simulink model "Hardware_testng_simulink_both"  (R2024b)
settings: Solver=ode1  StartTime=0.0  StopTime=15  FixedStep=0.005  RelTol=1e-3  EnableMultiTasking=on
undefined symbols (not defined in the file or in its folder): DiscIntNeverNeededParam, initialPose, maxAngularAcc, maxAngularVel, maxLinearAcc, maxLinearVel, poseTol, Ts, wps1
libraries: simulink_extras x12, stmnucleolib x12, simulink x4, hdlsllib x1, embmathops x1, robotcorelib x1
(part 1 of 2)
settings Model: ExtModeTrigDuration=10  Creator=ASUS  LastModifiedBy=Chhay
settings OptimizationCC: EnhancedBackFolding=on  PassReuseOutputArgsAs=Individual arguments  ZeroExternalMemoryAtStartup=off  ZeroInternalMemoryAtStartup=off  MaxStackSize=64  OptimizeBlockOrder=speed  DifferentSizesBufferReuse=on  OptimizationCustomize=off  EfficientTunableParamExpr=on
settings DebuggingCC: ParameterTunabilityLossMsg=error
settings HardwareCC: ProdBitPerPointer=32  ProdBitPerSizeT=32  ProdBitPerPtrDiffT=32  ProdLargestAtomicInteger=Long  ProdLargestAtomicFloat=Double  ProdWordSize=32  ProdLongLongMode=on  ProdHWDeviceType=ARM Compatible->ARM Cortex
settings SFSimCC: MATLABDynamicMemAlloc=off
settings RTWCC: Description=Embedded Coder  SystemTargetFile=ert.tlc  HardwareBoard=STM32 Nucleo H743ZI2  TemplateMakefile=ert_default_tmf  Toolchain=GNU Tools for ARM Embedded Processors  GPUComputeCapability=3.5
settings CodeAppCC: ForceParamTrailComments=on  IgnoreCustomStorageClasses=off  OperatorAnnotations=on  SimulinkDataObjDesc=on  SFDataObjDesc=on  InsertBlockDesc=on
settings ERTTargetCC: SupportContinuousTime=on  SupportVariableSizeSignals=on  ExtModeTransport=3  ExtModeStaticAlloc=on  ExtModeStaticAllocSize=2000  ExtModeMexFile=ext_xcp  ExtModeMexArgs=1 6 115200  ExtModeIntrfLevel=Level2 - Open  InlinedParameterPlacement=Hierarchical  RootIOFormat=Structure reference  DynamicArrayContainerType=coder::array

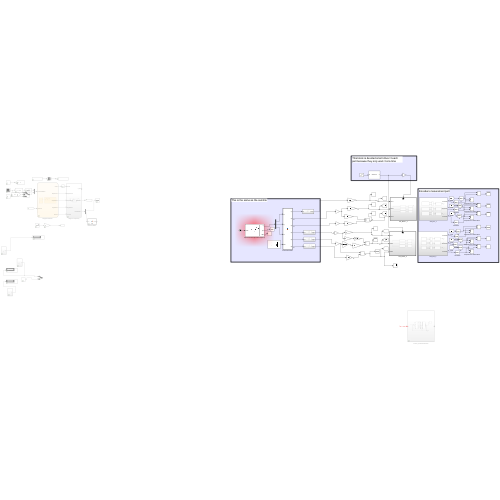
[thumbnail: Simulink's stored preview of the top-level diagram]
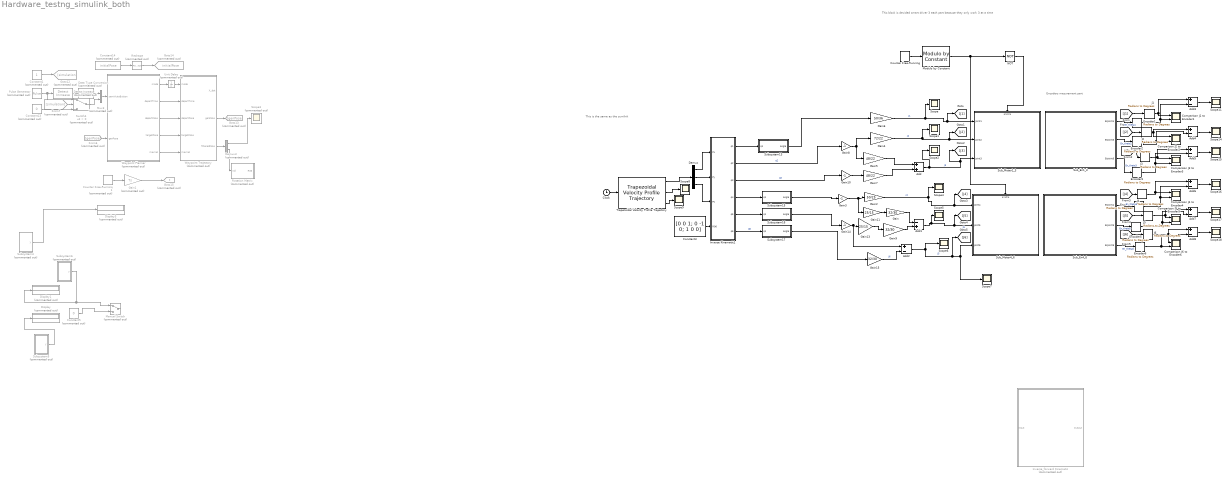
== system Hardware_testng_simulink_both ==
  note: Encoders mesurement part
  note: This block is devided smart driver 3 each part because they only work 3 at a time
  note: This is the same as the sumlink
  Add : Sum
  Add1 : Sum  Inputs=-+
  Add{2..8} (7 alike) : Sum  Inputs=+-
  Clock : Clock
  Comparison J1 to Encoder1 : Scope  NumInputPorts=2
  Comparison J2 to Encoder2 : Scope  NumInputPorts=2
  Comparison J3 to Encoder3 : Scope  NumInputPorts=2
  Comparison J4 to Encoder4 : Scope  NumInputPorts=2
  Comparison J5 to Encoder5 : Scope  NumInputPorts=2
  Comparison J6 to Encoder6 : Scope  NumInputPorts=2
  Constant1 : Constant  Commented=on
  Constant13 : Constant  Commented=on  Value=0
  Constant14 : Constant  Commented=on  Value=initialPose
  Constant3 : Constant  Value=[0 0 1; 0 -1 0; 1 0 0]
  Constant5 : Constant  Commented=on  Value=0
  Counter Free-Running : hdlsllib/Sources/Counter Free-Running  NumBits=16  tsamp=-1
  Counter Free-Running1 : simulink/Sources/Counter Free-Running  Commented=on  NumBits=16  tsamp=-1
  Data Type Conversion : DataTypeConversion  Commented=on  OutDataTypeStr=double  SaturateOnIntegerOverflow=off  RndMeth=Floor
  Demux : Demux  Outputs=3
  Demux3 : Demux  Commented=on  Outputs=[3,1]
  Detect Increase : simulink/Logic and Bit Operations/Detect Increase  Commented=on  vinit=0.0  OutDataTypeStr=boolean
  Display : Display  Commented=on
  Display1 : Display  Commented=on
  Display3 : Display  Commented=on
  Encoder{1..6} (6 alike) : simulink_extras/Transformations/Radians to Degrees
  From6 : From  Commented=on  GotoTag=genPose
  From7 : From  Commented=on  GotoTag=simulation
  Gain : Gain  Gain=32/30
  Gain1 : Gain  Commented=on  Gain=Ts  OutDataTypeStr=double
  Gain{3,8,10,14} (4 alike) : Gain  Gain=-1
  Gain11 : Gain  Gain=25/15
  Gain13 : Gain  Gain=25/15
  Gain15 : Gain  Gain=32/30
  Gain2 : Gain  Gain=50/25
  Gain4 : Gain  Gain=72/22
  Gain5 : Gain  Gain=48/22
  Gain6 : Gain  Gain=50/36  OutDataTypeStr=Inherit: Same as input
  Gain7 : Gain  Gain=48/22
  Gain9 : Gain  Gain=32/30
  Goto12 : Goto  Commented=on  GotoTag=simulation
  Goto13 : Goto  Commented=on  GotoTag=genPose
  Goto14 : Goto  Commented=on  GotoTag=initialPose  TagVisibility=global
  Goto15 : Goto  Commented=on  GotoTag=t  TagVisibility=global
  Inverse Kinematic1 : MATLAB Function  TreatAsAtomicUnit=on
  Inverse_forward Kinematic : Subsystem  Commented=on
  J{1..6} (6 alike) : simulink_extras/Transformations/Radians to Degrees
  Manual Switch : ManualSwitch  Commented=on
  Modulo by Constant : embmathops/Modulo by Constant  Denominator=2  SimulateUsing=Code generation
      settings: LibrarySourceBlock=embeddedMathLib/Modulo by Constant
  Mux3 : Mux  Commented=on  Inputs=2
  NOT : Logic  Operator=NOT  IconShape=distinctive  AllPortsSameDT=off  OutDataTypeStr=boolean
  Pulse Generator : DiscretePulseGenerator  Commented=on  PulseType=Time based  Period=30  PulseWidth=5  PhaseDelay=5
  Reshape : Reshape  Commented=on  OutputDimensionality=Column vector (2-D)
  Rotation Matrix : MATLAB Function  Commented=on  TreatAsAtomicUnit=on
  Scope{,1..2,4..9,11,14..18} (15 alike) : Scope
  Scope3 : Scope  Commented=on
  Sub_En1_3 : Subsystem
  Sub_En4_6 : Subsystem
  Sub_Moter1_3 : Subsystem
  Sub_Moter4_6 : Subsystem
  Subsystem13 : Subsystem
  Subsystem15 : Subsystem
  Subsystem16 : Subsystem
  Subsystem17 : Subsystem
  Subsystem4 : Subsystem  Commented=on
  Subsystem5 : Subsystem  Commented=on
  Subsystem6 : Subsystem  Commented=on
  Switch4 : Switch  Commented=on  Criteria=u2 > Threshold  SaturateOnIntegerOverflow=off  InputSameDT=off
  Trapezoidal Velocity Profile Trajectory : robotcorelib/Trapezoidal Velocity Profile Trajectory  WaypointSource=Internal  Waypoints=Way4  NumParams=1  Parameter1=End Time  Parameter2=End Time  ParameterSource=Internal  PeakVelocity=[ 2; 2 ]  Acceleration=[ 1; 2 ]  EndTime=2  AccelTime=[ 1; 2 ]  SimulateUsing=Interpreted execution
  Unit Delay : UnitDelay  Commented=on  SampleTime=-1  HasFrameUpgradeWarning=on
  Waypoint Planner : Stateflow chart  Commented=on  TreatAsAtomicUnit=on
      settings: PortSchema="{\"entries\":[{\"content\":{\"sides\":[{\"content\":{\"connectorIds\":[\"In2\",\"In1\"]},\"type\":\"ConnectorPlacement.EquallySpacedRectSide\",\"uuid\":\"2f7816bf-e041-4d80-a35c-f5abf025ca4f\"},{\"content\":{\"connectorIds\":[\"Out5\",\"Out1\",\"Out2\",\"Out3\",\"Out4\"],\"side\":\"RIGHT\"},\"type\":\"ConnectorPlacement.EquallySpacedRectSide\",\"uuid\":\"030a9877-c717-421f-9736-0adf27f6f35f\"},{\"content\":{\"side\":\"TOP\"},\"type\":\"ConnectorPlacement.EquallySpacedRectSide\",\"uuid\":\"ba023d22-bb45-4b84-a72f-1110f01393be\"}]},\"type\":\"ConnectorPlacement.EquallySpacedConnector\",\"uuid\":\"d2a85391-dfa2-4741-8917-4ca0c8ef44a5\"}],\"packageUris\":[\"http://schema.mathworks.com/mf0/Connector/R2020b\"],\"version\":\"1.0\"}"
  Waypoint Trajectory : Subsystem  Commented=on
  wires:
  Counter Free-Running/1 -> Modulo by Constant/1
  Modulo by Constant/1 -> NOT/1, Sub_Moter4_6/Enable
  NOT/1 -> Sub_Moter1_3/Enable
  Gain/1 -> Add1/1
  Gain2/1 -> [J4], Sub_Moter4_6/1(joint4), Scope4/1  "J4"
  Gain6/1 -> Scope/1, Sub_Moter1_3/1(Joint1), [J1]  "J1"
  Gain5/1 -> Add/1
  Gain7/1 -> Add/2
  Sub_En1_3/1(EnJoint4) -> Encoder1/1  "En_theta1"
  Sub_En1_3/2(EnJoint5) -> Encoder2/1  "En_theta2"
  Sub_En1_3/3(EnJoint6) -> Encoder3/1  "En_theta3"
  Sub_En4_6/2(EnJoint5) -> Encoder5/1  "En_theta5"
  Sub_En4_6/3(EnJoint6) -> Encoder6/1  "En_theta6"
  Gain4/1 -> Sub_Moter1_3/2(Joint2), [J2], Scope1/1  "J2"
  Gain15/1 -> Add2/2  "J6"
  Gain13/1 -> Gain9/1
  Add/1 -> Sub_Moter1_3/3(Joint3), [J3], Scope2/1  "J3"
  Add1/1 -> Scope5/1, [J5], Sub_Moter4_6/2(Joint5)  "J5"
  Gain9/1 -> Add1/2
  Gain11/1 -> Gain/1
  [J1] -> J1/1
  [J2] -> J2/1
  [J3] -> J3/1
  [J5] -> J5/1
  [J6] -> J6/1
  [J4] -> J4/1
  Sub_En4_6/1(EnJoint4) -> Encoder4/1  "En_theta3"
  Add3/1 -> Scope11/1
  Add4/1 -> Scope14/1
  Add5/1 -> Scope15/1
  Add6/1 -> Scope16/1
  Add7/1 -> Scope17/1
  Add8/1 -> Scope18/1
  Gain14/1 -> Add2/1, Gain13/1
  Gain8/1 -> Gain5/1, Gain4/1
  Gain10/1 -> Gain7/1
  Subsystem16/1(angle) -> Gain14/1
  Subsystem13/1(angle) -> Gain6/1
  Subsystem15/1(angle) -> Gain3/1
  Encoder6/1 -> Add8/2, Comparison J6 to Encoder6/2
  J6/1 -> Add8/1, Comparison J6 to Encoder6/1
  Encoder5/1 -> Add7/2, Comparison J5 to Encoder5/2
  J5/1 -> Add7/1, Comparison J5 to Encoder5/1
  Encoder4/1 -> Add6/2, Comparison J4 to Encoder4/2
  J4/1 -> Add6/1, Comparison J4 to Encoder4/1
  Encoder3/1 -> Add5/2, Comparison J3 to Encoder3/2
  J3/1 -> Add5/1, Comparison J3 to Encoder3/1
  Encoder2/1 -> Add4/2, Comparison J2 to Encoder2/2
  J2/1 -> Comparison J2 to Encoder2/1, Add4/1
  Encoder1/1 -> Add3/2, Comparison J1 to Encoder1/2
  J1/1 -> Comparison J1 to Encoder1/1, Add3/1
  Subsystem17/1(angle) -> Gain15/1
  Add2/1 -> Scope6/1, Scope7/1, Sub_Moter4_6/3(Joint6), [J6]  "J5"
  Switch4/1 -> Mux3/2
  Unit Delay/1 -> Waypoint Trajectory/1(mode)
  Waypoint Trajectory/3(filteredPose) -> Demux3/1
  Reshape/1 -> Goto14/1
  From7/1 -> Switch4/2
  Waypoint Planner/2(departPose) -> Waypoint Trajectory/3(departPose)
  Demux3/1 -> Scope3/1
  Waypoint Trajectory/2(genPose) -> Goto13/1
  Waypoint Planner/3(targetPose) -> Waypoint Trajectory/4(targetPose)
  Constant13/1 -> Switch4/3
  Waypoint Planner/5(mode) -> Unit Delay/1
  Counter Free-Running1/1 -> Gain1/1
  Data Type Conversion/1 -> Mux3/1
  Waypoint Planner/1(departTime) -> Waypoint Trajectory/2(departTime)
  Inverse Kinematic1/6(q6) -> Subsystem17/1(q1)  "q6"
  Detect Increase/1 -> Data Type Conversion/1
  Demux3/2 -> Rotation Matrix/1(roll)
  Gain1/1 -> Goto15/1
  Constant1/1 -> Goto12/1
  From6/1 -> Waypoint Planner/1(genPose)
  Inverse Kinematic1/2(q2) -> Gain8/1  "q2"
  Constant14/1 -> Reshape/1
  Inverse Kinematic1/4(q4) -> Subsystem15/1(q1)
  Pulse Generator/1 -> Switch4/1, Detect Increase/1
  Inverse Kinematic1/5(q5) -> Subsystem16/1(q1)
  Inverse Kinematic1/1(q1) -> Subsystem13/1(q1)
  Mux3/1 -> Waypoint Planner/2(semiAutoButton)
  Inverse Kinematic1/3(q3) -> Gain10/1  "q3"
  Waypoint Planner/4(maxVel) -> Waypoint Trajectory/5(maxVel)
  ? -> Inverse_forward Kinematic/1(Input)
  Gain3/1 -> Gain11/1, Gain2/1
  Constant3/1 -> Inverse Kinematic1/4(R06)
  Trapezoidal Velocity Profile Trajectory/1 -> Demux/1
  Clock/1 -> Trapezoidal Velocity Profile Trajectory/1
  Subsystem4/1(y) -> Display3/1
  Subsystem5/1(y) -> Display/1
  Demux/1 -> Inverse Kinematic1/1(Px)
  Constant5/1 -> Manual Switch/2
  Subsystem6/1(y) -> Manual Switch/1, Display1/1
  Demux/2 -> Inverse Kinematic1/2(Py)
  Demux/3 -> Inverse Kinematic1/3(Pz)
  Trapezoidal Velocity Profile Trajectory/2 -> Scope8/1
  Trapezoidal Velocity Profile Trajectory/3 -> Scope9/1

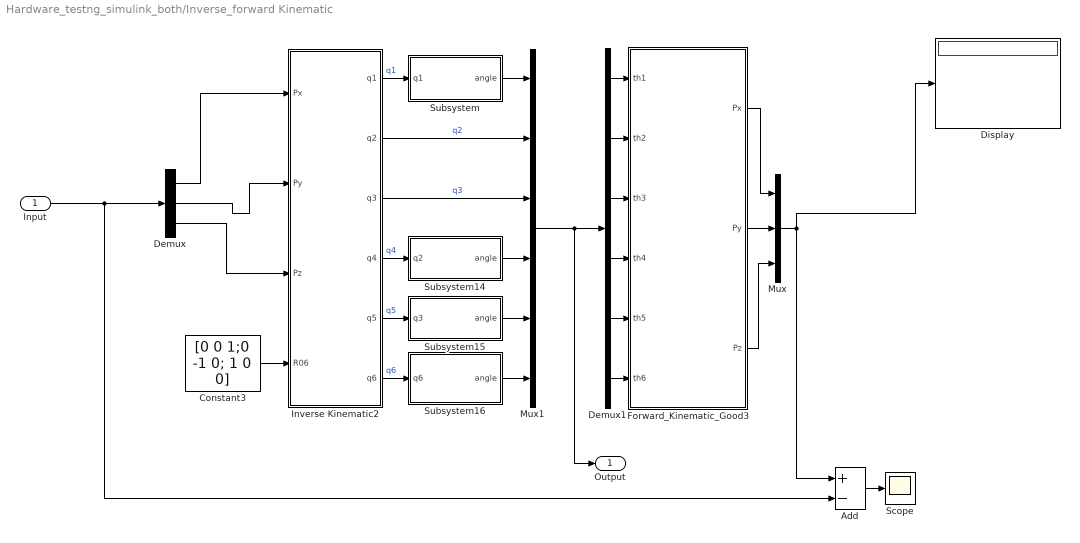
== system Hardware_testng_simulink_both/Inverse_forward Kinematic ==
  Input : Inport
  Add : Sum  Inputs=+-
  Constant3 : Constant  Value=[0 0 1;0 -1 0; 1 0 0]
  Demux : Demux  Outputs=3
  Demux1 : Demux  Outputs=6
  Display : Display
  Forward_Kinematic_Good3 : MATLAB Function  TreatAsAtomicUnit=on
  Inverse Kinematic2 : MATLAB Function  TreatAsAtomicUnit=on
  Mux : Mux  Inputs=3
  Mux1 : Mux  Inputs=6
  Scope : Scope
  Subsystem : Subsystem
  Subsystem14 : Subsystem
  Subsystem15 : Subsystem
  Subsystem16 : Subsystem
  Output : Outport
  wires:
  Forward_Kinematic_Good3/1(Px) -> Mux/1
  Demux/1 -> Inverse Kinematic2/1(Px)
  Forward_Kinematic_Good3/3(Pz) -> Mux/3
  Inverse Kinematic2/6(q6) -> Subsystem16/1(q6)  "q6"
  Forward_Kinematic_Good3/2(Py) -> Mux/2
  Inverse Kinematic2/4(q4) -> Subsystem14/1(q2)  "q4"
  Inverse Kinematic2/5(q5) -> Subsystem15/1(q3)  "q5"
  Constant3/1 -> Inverse Kinematic2/4(R06)
  Demux/2 -> Inverse Kinematic2/2(Py)
  Mux/1 -> Add/1, Display/1
  Demux/3 -> Inverse Kinematic2/3(Pz)
  Inverse Kinematic2/1(q1) -> Subsystem/1(q1)  "q1"
  Input/1 -> Add/2, Demux/1
  Subsystem15/1(angle) -> Mux1/5
  Subsystem/1(angle) -> Mux1/1
  Subsystem14/1(angle) -> Mux1/4
  Subsystem16/1(angle) -> Mux1/6
  Inverse Kinematic2/3(q3) -> Mux1/3  "q3"
  Inverse Kinematic2/2(q2) -> Mux1/2  "q2"
  Mux1/1 -> Output/1, Demux1/1
  Demux1/1 -> Forward_Kinematic_Good3/1(th1)
  Demux1/2 -> Forward_Kinematic_Good3/2(th2)
  Demux1/3 -> Forward_Kinematic_Good3/3(th3)
  Demux1/4 -> Forward_Kinematic_Good3/4(th4)
  Demux1/5 -> Forward_Kinematic_Good3/5(th5)
  Demux1/6 -> Forward_Kinematic_Good3/6(th6)
  Add/1 -> Scope/1

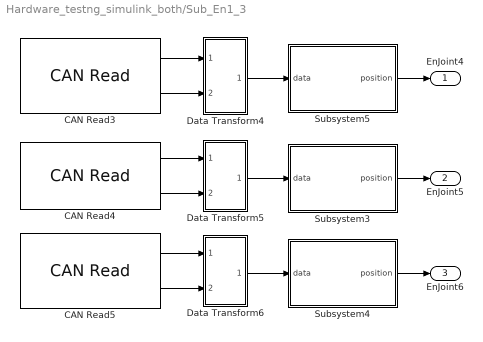
== system Hardware_testng_simulink_both/Sub_En1_3 ==
  CAN Read3 : stmnucleolib/CAN Read  CANModule=0  Identifier=Standard (11-bit identifier)  MsgId=254  MsgLen=8  RemoteFrame=off  OutputStatus=on  SampleTime=-1
      settings: LibrarySourceBlock=stmnucleoh7lib/CAN Read  DataFormat=Raw Data
  CAN Read4 : stmnucleolib/CAN Read  CANModule=0  Identifier=Standard (11-bit identifier)  MsgId=253  MsgLen=8  RemoteFrame=off  OutputStatus=on  SampleTime=-1
      settings: LibrarySourceBlock=stmnucleoh7lib/CAN Read  DataFormat=Raw Data
  CAN Read5 : stmnucleolib/CAN Read  CANModule=0  Identifier=Standard (11-bit identifier)  MsgId=252  MsgLen=8  RemoteFrame=off  OutputStatus=on  SampleTime=-1
      settings: LibrarySourceBlock=stmnucleoh7lib/CAN Read  DataFormat=Raw Data
  Data Transform4 : Subsystem
  Data Transform5 : Subsystem
  Data Transform6 : Subsystem
  Subsystem3 : Subsystem
  Subsystem4 : Subsystem
  Subsystem5 : Subsystem
  EnJoint4 : Outport
  EnJoint5 : Outport  Port=2
  EnJoint6 : Outport  Port=3
  wires:
  Subsystem3/1(position) -> EnJoint5/1
  Data Transform4/1(Data_T) -> Subsystem5/1(data)
  CAN Read5/1 -> Data Transform6/1(In1)
  CAN Read3/2 -> Data Transform4/2(In2)
  CAN Read5/2 -> Data Transform6/2(In2)
  CAN Read4/1 -> Data Transform5/1(In1)
  CAN Read3/1 -> Data Transform4/1(In1)
  Subsystem5/1(position) -> EnJoint4/1
  Data Transform6/1(Data_T) -> Subsystem4/1(data)
  Data Transform5/1(Data_T) -> Subsystem3/1(data)
  Subsystem4/1(position) -> EnJoint6/1
  CAN Read4/2 -> Data Transform5/2(In2)

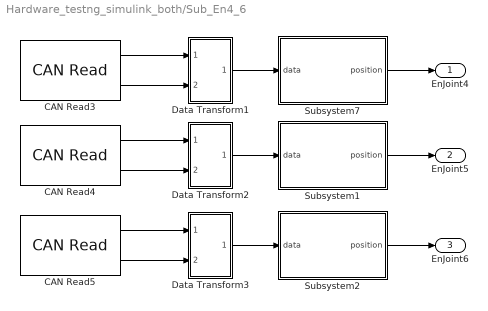
== system Hardware_testng_simulink_both/Sub_En4_6 ==
  CAN Read3 : stmnucleolib/CAN Read  CANModule=0  Identifier=Standard (11-bit identifier)  MsgId=251  MsgLen=8  RemoteFrame=off  OutputStatus=on  SampleTime=-1
      settings: LibrarySourceBlock=stmnucleoh7lib/CAN Read  DataFormat=Raw Data
  CAN Read4 : stmnucleolib/CAN Read  CANModule=0  Identifier=Standard (11-bit identifier)  MsgId=250  MsgLen=8  RemoteFrame=off  OutputStatus=on  SampleTime=-1
      settings: LibrarySourceBlock=stmnucleoh7lib/CAN Read  DataFormat=Raw Data
  CAN Read5 : stmnucleolib/CAN Read  CANModule=0  Identifier=Standard (11-bit identifier)  MsgId=249  MsgLen=8  RemoteFrame=off  OutputStatus=on  SampleTime=-1
      settings: LibrarySourceBlock=stmnucleoh7lib/CAN Read  DataFormat=Raw Data
  Data Transform1 : Subsystem
  Data Transform2 : Subsystem
  Data Transform3 : Subsystem
  Subsystem1 : Subsystem
  Subsystem2 : Subsystem
  Subsystem7 : Subsystem
  EnJoint4 : Outport
  EnJoint5 : Outport  Port=2
  EnJoint6 : Outport  Port=3
  wires:
  CAN Read3/2 -> Data Transform1/2(In2)
  Subsystem2/1(position) -> EnJoint6/1
  CAN Read4/2 -> Data Transform2/2(In2)
  Data Transform1/1(Data_T) -> Subsystem7/1(data)
  CAN Read4/1 -> Data Transform2/1(In1)
  Data Transform2/1(Data_T) -> Subsystem1/1(data)
  Subsystem1/1(position) -> EnJoint5/1
  CAN Read5/2 -> Data Transform3/2(In2)
  Subsystem7/1(position) -> EnJoint4/1
  CAN Read5/1 -> Data Transform3/1(In1)
  CAN Read3/1 -> Data Transform1/1(In1)
  Data Transform3/1(Data_T) -> Subsystem2/1(data)

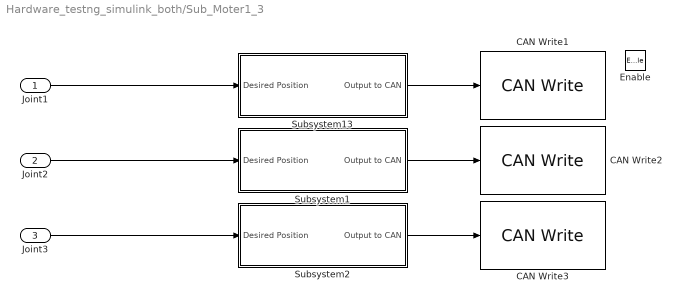
== system Hardware_testng_simulink_both/Sub_Moter1_3 ==
  Joint1 : Inport
  Joint2 : Inport  Port=2
  Joint3 : Inport  Port=3
  Enable : EnablePort
  CAN Write1 : stmnucleolib/CAN Write  CANModule=0  Identifier=Standard (11-bit identifier)  MsgId=1  MsgLen=8  RemoteFrame=off  OutputStatus=off
      settings: LibrarySourceBlock=stmnucleoh7lib/CAN Write  DataFormat=Raw Data
  CAN Write2 : stmnucleolib/CAN Write  CANModule=0  Identifier=Standard (11-bit identifier)  MsgId=2  MsgLen=8  RemoteFrame=off  OutputStatus=off
      settings: LibrarySourceBlock=stmnucleoh7lib/CAN Write  DataFormat=Raw Data
  CAN Write3 : stmnucleolib/CAN Write  CANModule=0  Identifier=Standard (11-bit identifier)  MsgId=3  MsgLen=8  RemoteFrame=off  OutputStatus=off
      settings: LibrarySourceBlock=stmnucleoh7lib/CAN Write  DataFormat=Raw Data
  Subsystem1 : Subsystem
  Subsystem13 : Subsystem
  Subsystem2 : Subsystem
  wires:
  Subsystem2/1(Output to CAN) -> CAN Write3/1
  Subsystem1/1(Output to CAN) -> CAN Write2/1
  Joint2/1 -> Subsystem1/1(Desired Position)
  Joint1/1 -> Subsystem13/1(Desired Position)
  Subsystem13/1(Output to CAN) -> CAN Write1/1
  Joint3/1 -> Subsystem2/1(Desired Position)

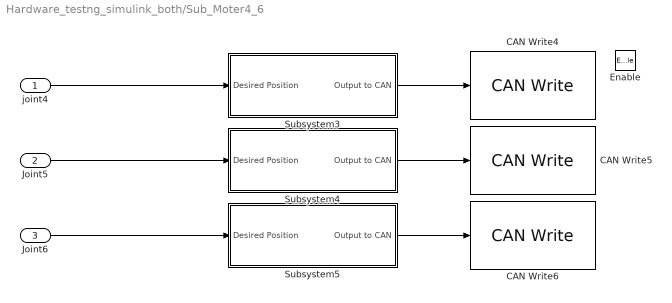
== system Hardware_testng_simulink_both/Sub_Moter4_6 ==
  joint4 : Inport
  Joint5 : Inport  Port=2
  Joint6 : Inport  Port=3
  Enable : EnablePort
  CAN Write4 : stmnucleolib/CAN Write  CANModule=0  Identifier=Standard (11-bit identifier)  MsgId=4  MsgLen=8  RemoteFrame=off  OutputStatus=off
      settings: LibrarySourceBlock=stmnucleoh7lib/CAN Write  DataFormat=Raw Data
  CAN Write5 : stmnucleolib/CAN Write  CANModule=0  Identifier=Standard (11-bit identifier)  MsgId=5  MsgLen=8  RemoteFrame=off  OutputStatus=off
      settings: LibrarySourceBlock=stmnucleoh7lib/CAN Write  DataFormat=Raw Data
  CAN Write6 : stmnucleolib/CAN Write  CANModule=0  Identifier=Standard (11-bit identifier)  MsgId=6  MsgLen=8  RemoteFrame=off  OutputStatus=off
      settings: LibrarySourceBlock=stmnucleoh7lib/CAN Write  DataFormat=Raw Data
  Subsystem3 : Subsystem
  Subsystem4 : Subsystem
  Subsystem5 : Subsystem
  wires:
  Subsystem4/1(Output to CAN) -> CAN Write5/1
  Joint6/1 -> Subsystem5/1(Desired Position)
  Subsystem5/1(Output to CAN) -> CAN Write6/1
  Joint5/1 -> Subsystem4/1(Desired Position)
  Subsystem3/1(Output to CAN) -> CAN Write4/1
  joint4/1 -> Subsystem3/1(Desired Position)

== system Hardware_testng_simulink_both/Subsystem13 ==
  q1 : Inport
  Constant1 : Constant
  Define Relative angle1 : MATLAB Function  TreatAsAtomicUnit=on
  Ground : Ground
  Ground1 : Ground
  angle : Outport
  wires:
  Ground/1 -> Define Relative angle1/1(initialPose)
  Define Relative angle1/1(angle) -> angle/1
  Constant1/1 -> Define Relative angle1/4(status)
  Ground1/1 -> Define Relative angle1/2(reset_angle)
  q1/1 -> Define Relative angle1/3(rawangle)

== system Hardware_testng_simulink_both/Subsystem15 ==
  q1 : Inport
  Constant1 : Constant
  Define Relative angle1 : MATLAB Function  TreatAsAtomicUnit=on
  Ground : Ground
  Ground1 : Ground
  angle : Outport
  wires:
  Ground/1 -> Define Relative angle1/1(initialPose)
  Define Relative angle1/1(angle) -> angle/1
  Constant1/1 -> Define Relative angle1/4(status)
  Ground1/1 -> Define Relative angle1/2(reset_angle)
  q1/1 -> Define Relative angle1/3(rawangle)

== system Hardware_testng_simulink_both/Subsystem16 ==
  q1 : Inport
  Constant1 : Constant
  Define Relative angle1 : MATLAB Function  TreatAsAtomicUnit=on
  Ground : Ground
  Ground1 : Ground
  angle : Outport
  wires:
  q1/1 -> Define Relative angle1/3(rawangle)
  Ground1/1 -> Define Relative angle1/2(reset_angle)
  Constant1/1 -> Define Relative angle1/4(status)
  Define Relative angle1/1(angle) -> angle/1
  Ground/1 -> Define Relative angle1/1(initialPose)

== system Hardware_testng_simulink_both/Subsystem17 ==
  q1 : Inport
  Constant1 : Constant
  Define Relative angle : MATLAB Function  TreatAsAtomicUnit=on
  Ground : Ground
  Ground1 : Ground
  angle : Outport
  wires:
  Ground/1 -> Define Relative angle/1(initialPose)
  Define Relative angle/1(angle) -> angle/1
  Constant1/1 -> Define Relative angle/4(status)
  Ground1/1 -> Define Relative angle/2(reset_angle)
  q1/1 -> Define Relative angle/3(rawangle)

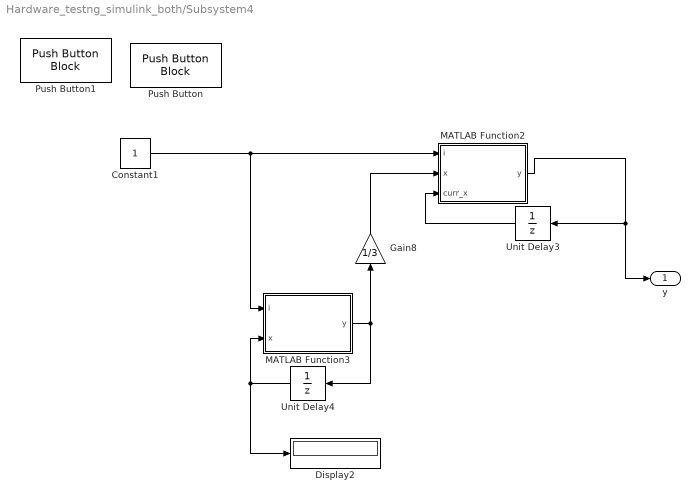
== system Hardware_testng_simulink_both/Subsystem4 ==
  Constant1 : Constant
  Display2 : Display
  Gain8 : Gain  Gain=1/3
  MATLAB Function2 : MATLAB Function  TreatAsAtomicUnit=on
  MATLAB Function3 : MATLAB Function  TreatAsAtomicUnit=on
  Push Button : PushButtonBlock  OffValue=1.000000
  Push Button1 : PushButtonBlock  OnValue=-1  OffValue=-1.000000
  Unit Delay3 : UnitDelay  SampleTime=-1  HasFrameUpgradeWarning=on
  Unit Delay4 : UnitDelay  SampleTime=-1  HasFrameUpgradeWarning=on
  y : Outport
  wires:
  Constant1/1 -> MATLAB Function2/1(i), MATLAB Function3/1(i)
  Gain8/1 -> MATLAB Function2/2(x)
  MATLAB Function3/1(y) -> Gain8/1, Unit Delay4/1
  MATLAB Function2/1(y) -> y/1, Unit Delay3/1
  Unit Delay4/1 -> Display2/1, MATLAB Function3/2(x)
  Unit Delay3/1 -> MATLAB Function2/3(curr_x)

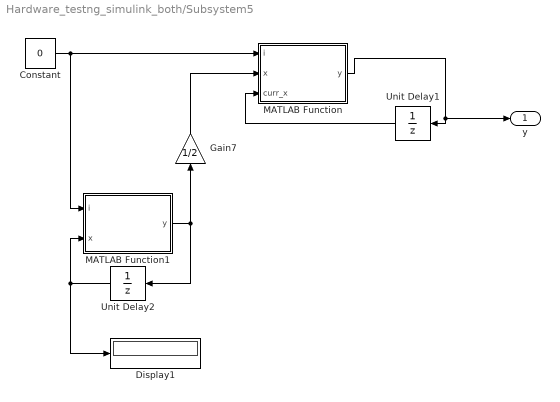
== system Hardware_testng_simulink_both/Subsystem5 ==
  Constant : Constant  Value=0
  Display1 : Display
  Gain7 : Gain  Gain=1/2
  MATLAB Function : MATLAB Function  TreatAsAtomicUnit=on
  MATLAB Function1 : MATLAB Function  TreatAsAtomicUnit=on
  Unit Delay1 : UnitDelay  SampleTime=-1  HasFrameUpgradeWarning=on
  Unit Delay2 : UnitDelay  SampleTime=-1  HasFrameUpgradeWarning=on
  y : Outport
  wires:
  Unit Delay1/1 -> MATLAB Function/3(curr_x)
  MATLAB Function1/1(y) -> Gain7/1, Unit Delay2/1
  MATLAB Function/1(y) -> y/1, Unit Delay1/1
  Constant/1 -> MATLAB Function/1(i), MATLAB Function1/1(i)
  Unit Delay2/1 -> Display1/1, MATLAB Function1/2(x)
  Gain7/1 -> MATLAB Function/2(x)

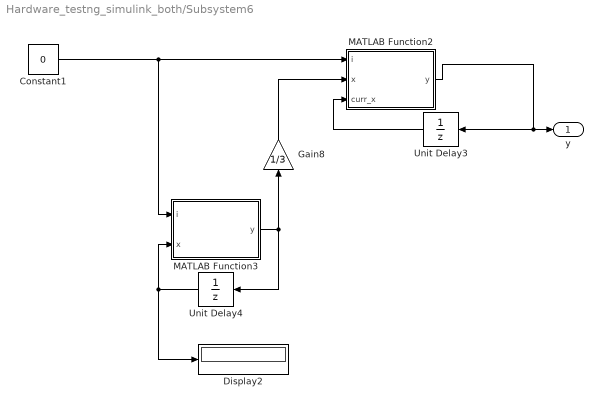
== system Hardware_testng_simulink_both/Subsystem6 ==
  Constant1 : Constant  Value=0
  Display2 : Display
  Gain8 : Gain  Gain=1/3
  MATLAB Function2 : MATLAB Function  TreatAsAtomicUnit=on
  MATLAB Function3 : MATLAB Function  TreatAsAtomicUnit=on
  Unit Delay3 : UnitDelay  SampleTime=-1  HasFrameUpgradeWarning=on
  Unit Delay4 : UnitDelay  SampleTime=-1  HasFrameUpgradeWarning=on
  y : Outport
  wires:
  Unit Delay4/1 -> Display2/1, MATLAB Function3/2(x)
  Constant1/1 -> MATLAB Function2/1(i), MATLAB Function3/1(i)
  Gain8/1 -> MATLAB Function2/2(x)
  MATLAB Function3/1(y) -> Gain8/1, Unit Delay4/1
  MATLAB Function2/1(y) -> y/1, Unit Delay3/1
  Unit Delay3/1 -> MATLAB Function2/3(curr_x)

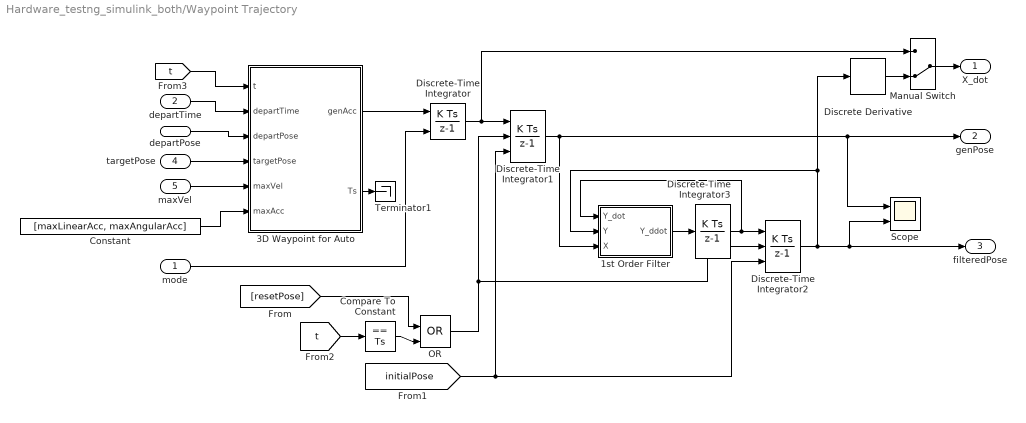
== system Hardware_testng_simulink_both/Waypoint Trajectory ==
  mode : Inport
  departTime : Inport  Port=2
  departPose : Inport  Port=3
  targetPose : Inport  Port=4
  maxVel : Inport  Port=5
  1st Order Filter : MATLAB Function  TreatAsAtomicUnit=on
  3D Waypoint for Auto : MATLAB Function  TreatAsAtomicUnit=on
  Compare To Constant : simulink/Logic and Bit Operations/Compare To Constant  relop===  const=Ts  OutDataTypeStr=boolean
  Constant : Constant  Value=[maxLinearAcc, maxAngularAcc]
  Discrete Derivative : simulink/Discrete/Discrete Derivative  gainval=1.0  ICPrevScaledInput=0.0  OutMin=[]  OutMax=[]  OutDataType=fixdt(1, 16)  OutScaling=2^-10  DoSatur=off
  Discrete-Time Integrator : DiscreteIntegrator  ExternalReset=falling  InitialCondition=[0;0;0;0]  SampleTime=-1  ICPrevOutput=DiscIntNeverNeededParam  ICPrevScaledInput=DiscIntNeverNeededParam
  Discrete-Time Integrator1 : DiscreteIntegrator  ExternalReset=rising  InitialConditionSource=external  InitialCondition=[0;0;0;0]  SampleTime=-1  ICPrevOutput=DiscIntNeverNeededParam  ICPrevScaledInput=DiscIntNeverNeededParam
  Discrete-Time Integrator2 : DiscreteIntegrator  ExternalReset=rising  InitialConditionSource=external  InitialCondition=[0;0;0;0]  SampleTime=-1  ICPrevOutput=DiscIntNeverNeededParam  ICPrevScaledInput=DiscIntNeverNeededParam
  Discrete-Time Integrator3 : DiscreteIntegrator  InitialCondition=[0;0;0;0]  SampleTime=-1  ICPrevOutput=DiscIntNeverNeededParam  ICPrevScaledInput=DiscIntNeverNeededParam
  Manual Switch : ManualSwitch  CurrentSetting=0
  OR : Logic  Operator=OR  IconShape=distinctive  AllPortsSameDT=off  OutDataTypeStr=boolean
  Scope : Scope  NumInputPorts=2
  Terminator1 : Terminator
  X_dot : Outport
  genPose : Outport  Port=2
  filteredPose : Outport  Port=3
  wires:
  Constant/1 -> 3D Waypoint for Auto/6(maxAcc)
  targetPose/1 -> 3D Waypoint for Auto/4(targetPose)
  maxVel/1 -> 3D Waypoint for Auto/5(maxVel)
  departTime/1 -> 3D Waypoint for Auto/2(departTime)
  [t] -> 3D Waypoint for Auto/1(t)
  departPose/1 -> 3D Waypoint for Auto/3(departPose)
  3D Waypoint for Auto/2(Ts) -> Terminator1/1
  Discrete-Time Integrator/1 -> Discrete-Time Integrator1/1, Manual Switch/1
  [t] -> Compare To Constant/1
  [resetPose] -> OR/1
  Compare To Constant/1 -> OR/2
  3D Waypoint for Auto/1(genAcc) -> Discrete-Time Integrator/1
  mode/1 -> Discrete-Time Integrator/2
  OR/1 -> Discrete-Time Integrator2/2, Discrete-Time Integrator1/2
  [initialPose] -> Discrete-Time Integrator1/3, Discrete-Time Integrator2/3
  Discrete-Time Integrator1/1 -> Scope/1, genPose/1, 1st Order Filter/3(X)
  1st Order Filter/1(Y_ddot) -> Discrete-Time Integrator3/1
  Discrete-Time Integrator2/1 -> Scope/2, filteredPose/1, Discrete Derivative/1, 1st Order Filter/2(Y)
  Discrete Derivative/1 -> Manual Switch/2
  Manual Switch/1 -> X_dot/1
  Discrete-Time Integrator3/1 -> 1st Order Filter/1(Y_dot), Discrete-Time Integrator2/1

== system Hardware_testng_simulink_both/Inverse_forward Kinematic/Subsystem ==
  q1 : Inport
  Constant1 : Constant
  Define Relative angle : MATLAB Function  TreatAsAtomicUnit=on
  Ground : Ground
  Ground1 : Ground
  angle : Outport
  wires:
  q1/1 -> Define Relative angle/3(rawangle)
  Ground1/1 -> Define Relative angle/2(reset_angle)
  Constant1/1 -> Define Relative angle/4(status)
  Define Relative angle/1(angle) -> angle/1
  Ground/1 -> Define Relative angle/1(initialPose)

== system Hardware_testng_simulink_both/Inverse_forward Kinematic/Subsystem14 ==
  q2 : Inport
  Constant1 : Constant
  Define Relative angle : MATLAB Function  TreatAsAtomicUnit=on
  Ground : Ground
  Ground1 : Ground
  angle : Outport
  wires:
  Ground/1 -> Define Relative angle/1(initialPose)
  Define Relative angle/1(angle) -> angle/1
  Constant1/1 -> Define Relative angle/4(status)
  Ground1/1 -> Define Relative angle/2(reset_angle)
  q2/1 -> Define Relative angle/3(rawangle)

== system Hardware_testng_simulink_both/Inverse_forward Kinematic/Subsystem15 ==
  q3 : Inport
  Constant1 : Constant
  Define Relative angle : MATLAB Function  TreatAsAtomicUnit=on
  Ground : Ground
  Ground1 : Ground
  angle : Outport
  wires:
  q3/1 -> Define Relative angle/3(rawangle)
  Ground1/1 -> Define Relative angle/2(reset_angle)
  Constant1/1 -> Define Relative angle/4(status)
  Define Relative angle/1(angle) -> angle/1
  Ground/1 -> Define Relative angle/1(initialPose)

== system Hardware_testng_simulink_both/Inverse_forward Kinematic/Subsystem16 ==
  q6 : Inport
  Constant1 : Constant
  Define Relative angle : MATLAB Function  TreatAsAtomicUnit=on
  Ground : Ground
  Ground1 : Ground
  angle : Outport
  wires:
  Ground/1 -> Define Relative angle/1(initialPose)
  Define Relative angle/1(angle) -> angle/1
  Constant1/1 -> Define Relative angle/4(status)
  Ground1/1 -> Define Relative angle/2(reset_angle)
  q6/1 -> Define Relative angle/3(rawangle)

== system Hardware_testng_simulink_both/Sub_En1_3/Data Transform4 ==
  In1 : Inport
  In2 : Inport  Port=2
  Enabled Subsystem1 : Subsystem  TreatAsAtomicUnit=on
  Data_T : Outport
  wires:
  Enabled Subsystem1/1(Input) -> Data_T/1
  In1/1 -> Enabled Subsystem1/1(In1)
  In2/1 -> Enabled Subsystem1/Enable

== system Hardware_testng_simulink_both/Sub_En1_3/Data Transform5 ==
  In1 : Inport
  In2 : Inport  Port=2
  Enabled Subsystem1 : Subsystem  TreatAsAtomicUnit=on
  Data_T : Outport
  wires:
  In2/1 -> Enabled Subsystem1/Enable
  In1/1 -> Enabled Subsystem1/1(In1)
  Enabled Subsystem1/1(Input) -> Data_T/1

== system Hardware_testng_simulink_both/Sub_En1_3/Data Transform6 ==
  In1 : Inport
  In2 : Inport  Port=2
  Enabled Subsystem1 : Subsystem  TreatAsAtomicUnit=on
  Data_T : Outport
  wires:
  Enabled Subsystem1/1(Input) -> Data_T/1
  In1/1 -> Enabled Subsystem1/1(In1)
  In2/1 -> Enabled Subsystem1/Enable

== system Hardware_testng_simulink_both/Sub_En1_3/Subsystem3 ==
  data : Inport
  MATLAB Function : MATLAB Function  TreatAsAtomicUnit=on
  Terminator : Terminator
  position : Outport
  wires:
  data/1 -> MATLAB Function/1(data)
  MATLAB Function/1(position) -> position/1
  MATLAB Function/2(speed) -> Terminator/1

== system Hardware_testng_simulink_both/Sub_En1_3/Subsystem4 ==
  data : Inport
  MATLAB Function : MATLAB Function  TreatAsAtomicUnit=on
  Terminator : Terminator
  position : Outport
  wires:
  MATLAB Function/2(speed) -> Terminator/1
  MATLAB Function/1(position) -> position/1
  data/1 -> MATLAB Function/1(data)

== system Hardware_testng_simulink_both/Sub_En1_3/Subsystem5 ==
  data : Inport
  MATLAB Function : MATLAB Function  TreatAsAtomicUnit=on
  Terminator : Terminator
  position : Outport
  wires:
  MATLAB Function/2(speed) -> Terminator/1
  MATLAB Function/1(position) -> position/1
  data/1 -> MATLAB Function/1(data)

== system Hardware_testng_simulink_both/Sub_En4_6/Data Transform1 ==
  In1 : Inport
  In2 : Inport  Port=2
  Enabled Subsystem1 : Subsystem  TreatAsAtomicUnit=on
  Data_T : Outport
  wires:
  Enabled Subsystem1/1(Input) -> Data_T/1
  In1/1 -> Enabled Subsystem1/1(In1)
  In2/1 -> Enabled Subsystem1/Enable

== system Hardware_testng_simulink_both/Sub_En4_6/Data Transform2 ==
  In1 : Inport
  In2 : Inport  Port=2
  Enabled Subsystem1 : Subsystem  TreatAsAtomicUnit=on
  Data_T : Outport
  wires:
  In2/1 -> Enabled Subsystem1/Enable
  In1/1 -> Enabled Subsystem1/1(In1)
  Enabled Subsystem1/1(Input) -> Data_T/1

== system Hardware_testng_simulink_both/Sub_En4_6/Data Transform3 ==
  In1 : Inport
  In2 : Inport  Port=2
  Enabled Subsystem1 : Subsystem  TreatAsAtomicUnit=on
  Data_T : Outport
  wires:
  Enabled Subsystem1/1(Input) -> Data_T/1
  In1/1 -> Enabled Subsystem1/1(In1)
  In2/1 -> Enabled Subsystem1/Enable

== system Hardware_testng_simulink_both/Sub_En4_6/Subsystem1 ==
  data : Inport
  MATLAB Function : MATLAB Function  TreatAsAtomicUnit=on
  Terminator : Terminator
  position : Outport
  wires:
  data/1 -> MATLAB Function/1(data)
  MATLAB Function/1(position) -> position/1
  MATLAB Function/2(speed) -> Terminator/1

== system Hardware_testng_simulink_both/Sub_En4_6/Subsystem2 ==
  data : Inport
  MATLAB Function : MATLAB Function  TreatAsAtomicUnit=on
  Terminator : Terminator
  position : Outport
  wires:
  MATLAB Function/2(speed) -> Terminator/1
  MATLAB Function/1(position) -> position/1
  data/1 -> MATLAB Function/1(data)

== system Hardware_testng_simulink_both/Sub_En4_6/Subsystem7 ==
  data : Inport
  MATLAB Function : MATLAB Function  TreatAsAtomicUnit=on
  Terminator : Terminator
  position : Outport
  wires:
  MATLAB Function/2(speed) -> Terminator/1
  MATLAB Function/1(position) -> position/1
  data/1 -> MATLAB Function/1(data)

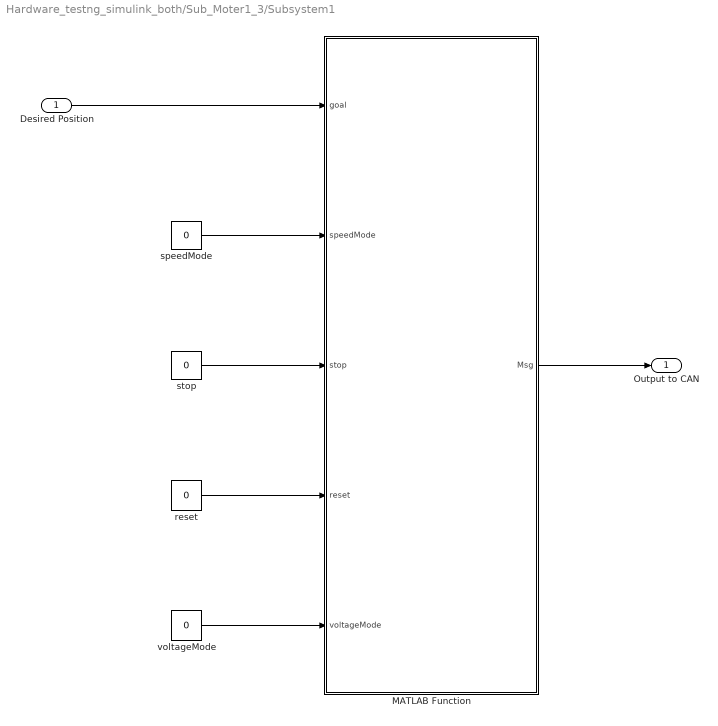
== system Hardware_testng_simulink_both/Sub_Moter1_3/Subsystem1 ==
  Desired Position : Inport
  MATLAB Function : MATLAB Function  TreatAsAtomicUnit=on
  reset : Constant  Value=0
  speedMode : Constant  Value=0  OutDataTypeStr=int16
  stop : Constant  Value=0  OutDataTypeStr=int16
  voltageMode : Constant  Value=0
  Output to CAN : Outport
  wires:
  reset/1 -> MATLAB Function/4(reset)
  Desired Position/1 -> MATLAB Function/1(goal)
  speedMode/1 -> MATLAB Function/2(speedMode)
  stop/1 -> MATLAB Function/3(stop)
  MATLAB Function/1(Msg) -> Output to CAN/1
  voltageMode/1 -> MATLAB Function/5(voltageMode)

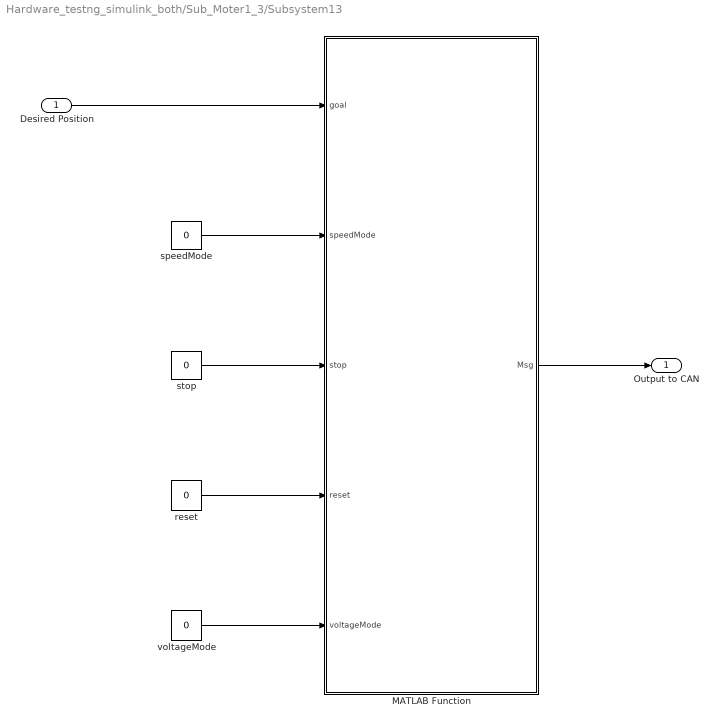
== system Hardware_testng_simulink_both/Sub_Moter1_3/Subsystem13 ==
  Desired Position : Inport
  MATLAB Function : MATLAB Function  TreatAsAtomicUnit=on
  reset : Constant  Value=0
  speedMode : Constant  Value=0  OutDataTypeStr=int16
  stop : Constant  Value=0  OutDataTypeStr=int16
  voltageMode : Constant  Value=0
  Output to CAN : Outport
  wires:
  voltageMode/1 -> MATLAB Function/5(voltageMode)
  MATLAB Function/1(Msg) -> Output to CAN/1
  stop/1 -> MATLAB Function/3(stop)
  speedMode/1 -> MATLAB Function/2(speedMode)
  Desired Position/1 -> MATLAB Function/1(goal)
  reset/1 -> MATLAB Function/4(reset)

== system Hardware_testng_simulink_both/Sub_Moter1_3/Subsystem2 ==
  Desired Position : Inport
  MATLAB Function : MATLAB Function  TreatAsAtomicUnit=on
  reset : Constant  Value=0
  speedMode : Constant  Value=0  OutDataTypeStr=int16
  stop : Constant  Value=0  OutDataTypeStr=int16
  voltageMode : Constant  Value=0
  Output to CAN : Outport
  wires:
  voltageMode/1 -> MATLAB Function/5(voltageMode)
  MATLAB Function/1(Msg) -> Output to CAN/1
  stop/1 -> MATLAB Function/3(stop)
  speedMode/1 -> MATLAB Function/2(speedMode)
  Desired Position/1 -> MATLAB Function/1(goal)
  reset/1 -> MATLAB Function/4(reset)

== system Hardware_testng_simulink_both/Sub_Moter4_6/Subsystem3 ==
  Desired Position : Inport
  MATLAB Function : MATLAB Function  TreatAsAtomicUnit=on
  reset : Constant  Value=0
  speedMode : Constant  Value=0  OutDataTypeStr=int16
  stop : Constant  Value=0  OutDataTypeStr=int16
  voltageMode : Constant  Value=0
  Output to CAN : Outport
  wires:
  reset/1 -> MATLAB Function/4(reset)
  Desired Position/1 -> MATLAB Function/1(goal)
  speedMode/1 -> MATLAB Function/2(speedMode)
  stop/1 -> MATLAB Function/3(stop)
  MATLAB Function/1(Msg) -> Output to CAN/1
  voltageMode/1 -> MATLAB Function/5(voltageMode)

== system Hardware_testng_simulink_both/Sub_Moter4_6/Subsystem4 ==
  Desired Position : Inport
  MATLAB Function : MATLAB Function  TreatAsAtomicUnit=on
  reset : Constant  Value=0
  speedMode : Constant  Value=0  OutDataTypeStr=int16
  stop : Constant  Value=0  OutDataTypeStr=int16
  voltageMode : Constant  Value=0
  Output to CAN : Outport
  wires:
  voltageMode/1 -> MATLAB Function/5(voltageMode)
  MATLAB Function/1(Msg) -> Output to CAN/1
  stop/1 -> MATLAB Function/3(stop)
  speedMode/1 -> MATLAB Function/2(speedMode)
  Desired Position/1 -> MATLAB Function/1(goal)
  reset/1 -> MATLAB Function/4(reset)

== system Hardware_testng_simulink_both/Sub_Moter4_6/Subsystem5 ==
  Desired Position : Inport
  MATLAB Function : MATLAB Function  TreatAsAtomicUnit=on
  reset : Constant  Value=0
  speedMode : Constant  Value=0  OutDataTypeStr=int16
  stop : Constant  Value=0  OutDataTypeStr=int16
  voltageMode : Constant  Value=0
  Output to CAN : Outport
  wires:
  reset/1 -> MATLAB Function/4(reset)
  Desired Position/1 -> MATLAB Function/1(goal)
  speedMode/1 -> MATLAB Function/2(speedMode)
  stop/1 -> MATLAB Function/3(stop)
  MATLAB Function/1(Msg) -> Output to CAN/1
  voltageMode/1 -> MATLAB Function/5(voltageMode)

== system Hardware_testng_simulink_both/Sub_En1_3/Data Transform4/Enabled Subsystem1 ==
  In1 : Inport
  Enable : EnablePort
  Input : Outport
  wires:
  In1/1 -> Input/1

== system Hardware_testng_simulink_both/Sub_En1_3/Data Transform5/Enabled Subsystem1 ==
  In1 : Inport
  Enable : EnablePort
  Input : Outport
  wires:
  In1/1 -> Input/1

== system Hardware_testng_simulink_both/Sub_En1_3/Data Transform6/Enabled Subsystem1 ==
  In1 : Inport
  Enable : EnablePort
  Input : Outport
  wires:
  In1/1 -> Input/1

== system Hardware_testng_simulink_both/Sub_En4_6/Data Transform1/Enabled Subsystem1 ==
  In1 : Inport
  Enable : EnablePort
  Input : Outport
  wires:
  In1/1 -> Input/1

== system Hardware_testng_simulink_both/Sub_En4_6/Data Transform2/Enabled Subsystem1 ==
  In1 : Inport
  Enable : EnablePort
  Input : Outport
  wires:
  In1/1 -> Input/1

== system Hardware_testng_simulink_both/Sub_En4_6/Data Transform3/Enabled Subsystem1 ==
  In1 : Inport
  Enable : EnablePort
  Input : Outport
  wires:
  In1/1 -> Input/1

== matlab function Hardware_testng_simulink_both/Sub_Moter1_3/Subsystem13/MATLAB Function ==
  data: goal input; Msg output; speedMode input; stop input; reset input; voltageMode input
function Msg = fcn(goal, speedMode, stop, reset, voltageMode)
    Msg = uint8(zeros(8,1));

    Msg(1) = speedMode + stop * 2 + reset * 4 + voltageMode * 8;

    Msg(3:6) = typecast(single(goal), 'uint8');
end

== matlab function Hardware_testng_simulink_both/Sub_Moter1_3/Subsystem1/MATLAB Function ==
  data: goal input; Msg output; speedMode input; stop input; reset input; voltageMode input
function Msg = fcn(goal, speedMode, stop, reset, voltageMode)
    Msg = uint8(zeros(8,1));

    Msg(1) = speedMode + stop * 2 + reset * 4 + voltageMode * 8;

    Msg(3:6) = typecast(single(goal), 'uint8');
end

== matlab function Hardware_testng_simulink_both/Sub_Moter1_3/Subsystem2/MATLAB Function ==
  data: goal input; Msg output; speedMode input; stop input; reset input; voltageMode input
function Msg = fcn(goal, speedMode, stop, reset, voltageMode)
    Msg = uint8(zeros(8,1));

    Msg(1) = speedMode + stop * 2 + reset * 4 + voltageMode * 8;

    Msg(3:6) = typecast(single(goal), 'uint8');
end

== matlab function Hardware_testng_simulink_both/Sub_Moter4_6/Subsystem3/MATLAB Function ==
  data: goal input; Msg output; speedMode input; stop input; reset input; voltageMode input
function Msg = fcn(goal, speedMode, stop, reset, voltageMode)
    Msg = uint8(zeros(8,1));

    Msg(1) = speedMode + stop * 2 + reset * 4 + voltageMode * 8;

    Msg(3:6) = typecast(single(goal), 'uint8');
end

== matlab function Hardware_testng_simulink_both/Sub_Moter4_6/Subsystem4/MATLAB Function ==
  data: goal input; Msg output; speedMode input; stop input; reset input; voltageMode input
function Msg = fcn(goal, speedMode, stop, reset, voltageMode)
    Msg = uint8(zeros(8,1));

    Msg(1) = speedMode + stop * 2 + reset * 4 + voltageMode * 8;

    Msg(3:6) = typecast(single(goal), 'uint8');
end

== matlab function Hardware_testng_simulink_both/Sub_Moter4_6/Subsystem5/MATLAB Function ==
  data: goal input; Msg output; speedMode input; stop input; reset input; voltageMode input
function Msg = fcn(goal, speedMode, stop, reset, voltageMode)
    Msg = uint8(zeros(8,1));

    Msg(1) = speedMode + stop * 2 + reset * 4 + voltageMode * 8;

    Msg(3:6) = typecast(single(goal), 'uint8');
end

== matlab function Hardware_testng_simulink_both/Sub_En1_3/Subsystem3/MATLAB Function ==
  data: data input; position output; speed output
function [position, speed] = fcn(data)
    %#codegen
    position = zeros(1, 1, 'single');
    speed = zeros(1, 1, 'single');

    if numel(data) >= 8
        position = typecast(data(1:4), 'single');
        speed = typecast(data(5:8), 'single');
    end
end

== matlab function Hardware_testng_simulink_both/Sub_En4_6/Subsystem7/MATLAB Function ==
  data: data input; position output; speed output
function [position, speed] = fcn(data)
    %#codegen
    position = zeros(1, 1, 'single');
    speed = zeros(1, 1, 'single');

    if numel(data) >= 8
        position = typecast(data(1:4), 'single');
        speed = typecast(data(5:8), 'single');
    end
end

== matlab function Hardware_testng_simulink_both/Inverse_forward Kinematic/Forward_Kinematic_Good3 ==
  data: Px output; Py output; Pz output; th1 input; th2 input; th3 input; th4 input; th5 input; th6 input
function [Px,Py,Pz] = forward_kinematics(th1, th2, th3, th4, th5, th6)
% 
% %     Define DH parameters
%     l1 = 276/1000;  % Length of link 1
%     l2 = 305.94661/1000 ;
%     l3 = 154.46177/1000;
%     l4 =228.74688/1000;% Length of link 2
%     l5 = 68.15773/1000;
%     l6=41.47212/1000 ;   % Length of link 6
%     a= 82.4965/1000;
%old length all in mm
 l1=276;
l2=306;
a=79.75;
l3=160;
l4=227;
l5=70;
l6=38;
    % Compute DH transformation matrices
    A0 = dh_matrix(0    , 0     ,l1 , th1);   
    A1 = dh_matrix(0    ,-pi/2  ,0  , th2-pi/2);
    A2 = dh_matrix(l2   ,0      ,0  ,th3);
    A3 = dh_matrix(a    ,-pi/2  ,0  ,th4);
    A4 = dh_matrix(0    ,0      ,l3+l4 ,0);
    A4p= dh_matrix(0   ,pi/2   ,0  ,th5);
    A5 = dh_matrix(0    ,-pi/2  , 0 ,th6);
    A6 = dh_matrix(0    ,0      ,l5+l6 ,0);
    
    % Total forward matrix H
    A0_6 = ( A0*A1 * A2 * A3 * A4 * A4p * A5 * A6) ;
    R06 =(A0_6(1:3,1:3));
    A03=A0*A1*A2 ;
    R03=(A03(1:3,1:3));
    A3_6= A3*A4*A4p*A5*A6;
    R36=(A3_6(1:3,1:3));
  


    Px=A0_6(1,4);
    Py=A0_6(2,4);
    Pz=A0_6(3,4);

end
function A = dh_matrix(a , alpha ,d ,theta)
    A = [cos(theta)            , -sin(theta),           0       ,   a;
         cos(alpha)*sin(theta), cos(theta)*cos(alpha), -sin(alpha), -d*sin(alpha);
         sin(alpha)*sin(theta), sin(alpha)*cos(theta), cos(alpha), d*cos(alpha);
         0, 0, 0, 1];
end

== matlab function Hardware_testng_simulink_both/Inverse_forward Kinematic/Inverse Kinematic2 ==
  settings: updateMethod=DISCRETE
  data: Px input; q1 output; Py input; Pz input; q2 output; q3 output; q4 output; q5 output; q6 output; R06 input
function [q1, q2, q3, q4, q5, q6] = inverseKinematics(Px, Py, Pz, R06)
    % Define actual geometry parameters (in meters)
%     l1 = 276;        % Length of link 1
%     l2 = 305.94661;  % Length of link 2
%     l3 = 154.46177;  % Length of link 3
%     l4 = 228.74688;  % Length of link 4
%     l5 = 68.15773;   % Length of link 5 (offset)
%     l6 = 41.47212;   % Length of link 6 (end-effector)
%     a  = 82.4965;    % Offset a
%%Old length 
l1=276;
l2=306;
a=79.75;
l3=160;
l4=227;
l5=70;
l6=38;

%     R06=[0    0   1
%          0   -1   0
%          1    0   0];
    % Wrist position calculation
    O6=[Px,Py,Pz]';
    d6=l5+l6;
    OW = O6 - R06*[0;0;d6];
%     r13 = R06(1, 3);
%     r23 = R06(2, 3);
%     r33 = R06(3, 3);

    % Compute wrist position (compensating for the end-effector offset)
%     Pwx = Px - (l5 + l6) * r13;
%     Pwy = Py - (l5 + l6) * r23;
%     Pwz = Pz - (l5 + l6) * r33;
Pwx=OW(1); Pwy=OW(2);Pwz=OW(3);

    % Compute q1 directly from the wrist position
    q1 = atan2(Pwy, Pwx);

    % Convert wrist position to cylindrical coordinates
    r = sqrt(Pwx^2 + Pwy^2);
    %new code 
    h= Pwz-l1;
    % my code: h = Pwz - l1;

    % Intermediate calculations for q2 and q3
    s = sqrt(h^2 + r^2);
     alp = atan(h/r );
    w3 = l3 + l4;
    k3 = sqrt(a^2 + w3^2);
    %phi2
    beta = acos((l2^2 + s^2 - k3^2) / (2 * l2 * s));
   %gamma or phi3
    gamma = acos(( -s^2+l2^2+k3^2) / (2 * l2 * k3));
    Phi = atan(w3/a);
    

    % Target angles for q2 and q3
    q2 = pi/2- alp -beta ;
    q3 =  pi- gamma - Phi;
%     q3= -gamma-pi/2;

    % Compute R0_3 from q1, q2, q3
    R03 = [cos(q1)*cos(q2 + q3), -cos(q1)*sin(q2 + q3), -sin(q1);
           sin(q1)*cos(q2 + q3), -sin(q1)*sin(q2 + q3),  cos(q1);
           -sin(q2 + q3)       , -cos(q2 + q3)        , 0 ];
%     R03t=transpose(R03);

    % Compute R3_6 from the known R0_3 and R0_6
    R3_6 = R03.'* R06;

    % Extract elements from R3_6 for calculating q4, q5, q6
    s5c4 = -R3_6(1, 3);
    c5   = R3_6(2, 3);
    s5s4 = R3_6(3, 3);
    s5c6 = R3_6(2, 1);
    s5s6 = -R3_6(2, 2);

    % Joint angle q5
    % q5m = atan2(-sqrt(1 - c5^2), c5);
     q5p = atan2(-sqrt(1-c5^2),c5);
% q5=acos(c5)

    % Joint angles q4 and q6 based on the sign of q5
    %if q5m < q5p
    %    q5=q5m;
    %    q4 = atan2(s4s5, c4s5);
    %    q6 = atan2(s5s6, -s5c6);
    %else    
        q5=q5p;
        q4 = atan2(-s5s4, -s5c4);
        q6 = atan2(s5s6, -s5c6);
    
    %end
end

== matlab function Hardware_testng_simulink_both/Sub_En4_6/Subsystem1/MATLAB Function ==
  data: data input; position output; speed output
function [position, speed] = fcn(data)
    %#codegen
    position = zeros(1, 1, 'single');
    speed = zeros(1, 1, 'single');

    if numel(data) >= 8
        position = typecast(data(1:4), 'single');
        speed = typecast(data(5:8), 'single');
    end
end

== matlab function Hardware_testng_simulink_both/Sub_En4_6/Subsystem2/MATLAB Function ==
  data: data input; position output; speed output
function [position, speed] = fcn(data)
    %#codegen
    position = zeros(1, 1, 'single');
    speed = zeros(1, 1, 'single');

    if numel(data) >= 8
        position = typecast(data(1:4), 'single');
        speed = typecast(data(5:8), 'single');
    end
end

== matlab function Hardware_testng_simulink_both/Rotation Matrix ==
  data: roll input; R06 output
function R06 = fcn(roll)

yaw   = pi;
pitch = -pi/2;

Rx   = [1    0         0
        0   cos(roll)  -sin(roll)
        0   sin(roll)   cos(roll)];
Ry   = [cos(pitch)   0   sin(pitch)
           0         1      0
        -sin(pitch)  0   cos(pitch)];
Rz   = [cos(yaw)  -sin(yaw)   0
        sin(yaw)   cos(yaw)   0
          0           0       1];

R06  = Rz*Ry*Rx;

== matlab function Hardware_testng_simulink_both/Subsystem15/Define Relative angle1 ==
  settings: updateMethod=DISCRETE
  data: initialPose input; reset_angle input; rawangle input; angle output; status input
function angle = fcn(initialPose, reset_angle, rawangle, status)

% continuousangle is absolute angle
% angle is relative angle

persistent prevPsi2pi jump rawangle_0 set_angle
if isempty(prevPsi2pi)
    prevPsi2pi = 0; jump = 0; rawangle_0 = rawangle; set_angle = 0;
end

if abs(rawangle-prevPsi2pi) >  pi
    if rawangle > 0
        jump = jump - 1;
    else
        jump = jump + 1;
    end
end
prevPsi2pi = rawangle;

continuousangle = rawangle + jump*2*pi; % continuous value

if (status && ~set_angle), rawangle_0 = continuousangle; set_angle  = 1; end

if reset_angle, rawangle_0 = continuousangle; end

angle = continuousangle - rawangle_0 + initialPose;

== matlab function Hardware_testng_simulink_both/Subsystem16/Define Relative angle1 ==
  settings: updateMethod=DISCRETE
  data: initialPose input; reset_angle input; rawangle input; angle output; status input
function angle = fcn(initialPose, reset_angle, rawangle, status)

% continuousangle is absolute angle
% angle is relative angle

persistent prevPsi2pi jump rawangle_0 set_angle
if isempty(prevPsi2pi)
    prevPsi2pi = 0; jump = 0; rawangle_0 = rawangle; set_angle = 0;
end

if abs(rawangle-prevPsi2pi) >  pi
    if rawangle > 0
        jump = jump - 1;
    else
        jump = jump + 1;
    end
end
prevPsi2pi = rawangle;

continuousangle = rawangle + jump*2*pi; % continuous value

if (status && ~set_angle), rawangle_0 = continuousangle; set_angle  = 1; end

if reset_angle, rawangle_0 = continuousangle; end

angle = continuousangle - rawangle_0 + initialPose;

== matlab function Hardware_testng_simulink_both/Subsystem17/Define Relative angle ==
  settings: updateMethod=DISCRETE
  data: initialPose input; reset_angle input; rawangle input; angle output; status input
function angle = fcn(initialPose, reset_angle, rawangle, status)

% continuousangle is absolute angle
% angle is relative angle

persistent prevPsi2pi jump rawangle_0 set_angle
if isempty(prevPsi2pi)
    prevPsi2pi = 0; jump = 0; rawangle_0 = rawangle; set_angle = 0;
end

if abs(rawangle-prevPsi2pi) >  pi
    if rawangle > 0
        jump = jump - 1;
    else
        jump = jump + 1;
    end
end
if abs(rawangle-prevPsi2pi) >  pi/2 && abs(rawangle-prevPsi2pi) < pi
    if rawangle > 0
        jump = jump - 1/2;
    else
        jump = jump + 1/2;
    end
end

prevPsi2pi = rawangle;

continuousangle = rawangle + jump*2*pi; % continuous value

if (status && ~set_angle), rawangle_0 = continuousangle; set_angle  = 1; end

if reset_angle, rawangle_0 = continuousangle; end

angle = continuousangle - rawangle_0 + initialPose;

== stateflow chart Hardware_testng_simulink_both/Waypoint Planner ==
  state Semi_auto
    en: wps = zeros(4,20); mode = auto ;
    du:
    state Delay1
    state Goto_up
      en:
      percentage = 10;
      moving(wps);
    (default) -> Goto_up : {move = 0; stage = 1;
        | col = width(wps1);
        | wps(:,2:col+1) = wps1;
        | wps(:,1) = genPose;}
    Goto_up -> Delay1 [order 1] : [semiAutoButton(1) &&...
        |  semiAutoButton(2)==1]
        | {move=0;
        | col = width(wps1);
        | wps(:,2:col+1) = wps1;
        | wps(:,1) = genPose;}
    Delay1 -> Goto_up : [after(3,sec)]
    Goto_up -> Goto_up [order 2] : [norm(targetPose - genPose)...
        | <poseTol && move<col]
  state Manual
    en:
    man = 0; auto = 1;
    departPose = genPose; stage = 0;
    targetPose  = genPose + [0;0;0;0];
    lastShotAng = 0; psi_inc = initialPose(4);
    maxVel        = [maxLinearVel , maxAngularVel];
    du:
  state moving(wayPoints) [function]
    (default) -> (junction 92) : {move = move+1;
        | departTime = t;
        | traject = wayPoints(:,2:end) - wayPoints(:,1:end-1);
        | departPose = genPose;
        | aheadPoint = traject(:,move);
        | psi_inc        = psi_inc + aheadPoint(4);
        | targetPose  = genPose+aheadPoint;
        | targetPose(4) = psi_inc - lastShotAng;
        | maxVel(1)   = percentage/100*maxLinearVel;
        | dist              = norm(aheadPoint(1:3));
        | deltaT          = dist/maxVel(1);
        | maxVel(2)   = min(maxAngularVel,...
        |                              abs(aheadPoint(4)/deltaT));}
  (default) -> Manual
  Manual -> Semi_auto : [semiAutoButton(1) &&...
      |  semiAutoButton(2)==1]
  data: wayPoints function_input; departTime output; departPose output; targetPose output; maxVel output; genPose input; maxLinearVel parameter; semiAutoButton input; poseTol parameter; mode output; dist local; auto local; man local; move local; aheadPoint local; deltaT local; maxAngularVel parameter; initialPose parameter; percentage local; lastShotAng local; stage local; psi_inc local; wps local; col local; wps1 parameter; traject local
